simulink library "inp"  (R2021b)
settings: Solver=VariableStepAuto  StartTime=0.0  StopTime=10.0  RelTol=1e-3
undefined symbols (not defined in the file): C_TASK_5MS_S, FALSE, KINP_AcoreReadyToSlp_flg_ovrdflg, KINP_AcoreReadyToSlp_flg_ovrdval, KINP_AllowMovThd_OTA_enum_ovrdflg, KINP_AllowMovThd_OTA_enum_ovrdval, KINP_APSAngleTarget_Deg_ovrdflg, KINP_APSAngleTarget_Deg_ovrdval, KINP_APSDecReq_mps2_ovrdflg, KINP_APSDecReq_mps2_ovrdval, KINP_APSDecReqA_flg_ovrdflg, KINP_APSDecReqA_flg_ovrdval, KINP_APSDFLL_cm_ovrdflg, KINP_APSDFLL_cm_ovrdval, KINP_APSDFLR_cm_ovrdflg, KINP_APSDFLR_cm_ovrdval, KINP_APSDRLL_cm_ovrdflg, KINP_APSDRLL_cm_ovrdval, KINP_APSDRLR_cm_ovrdflg, KINP_APSDRLR_cm_ovrdval, KINP_APSExitCondition_enum_ovrdflg, KINP_APSExitCondition_enum_ovrdval, KINP_APSHWVer_enum_ovrdflg, KINP_APSHWVer_enum_ovrdval, KINP_APSProgressPCT_pct_ovrdflg, KINP_APSProgressPCT_pct_ovrdval, KINP_APSReq_enum_ovrdflg, KINP_APSReq_enum_ovrdval, KINP_APSRQDisplay_enum_ovrdflg, KINP_APSRQDisplay_enum_ovrdval, KINP_APSRqEPASCtrl_flg_ovrdflg, KINP_APSRqEPASCtrl_flg_ovrdval, KINP_APSShiftPosnReq_enum_ovrdval, KINP_APSShiftPosnReq_enum_ovrflg, KINP_APSSpeedCMD_kph_ovrdval, KINP_APSSpeedCMD_kph_ovrflg, KINP_APSStaSystem_enum_ovrdflg, KINP_APSStaSystem_enum_ovrdval, KINP_APSSWVer_enum_ovrdflg, KINP_APSSWVer_enum_ovrdval, KINP_APSVMCReqA_flg_ovrdval, KINP_APSVMCReqA_flg_ovrflg, KINP_APSVRqEPASCtrl_flg_ovrdflg, KINP_APSVRqEPASCtrl_flg_ovrdval, KINP_AuxBattVolmV_mV_ovrdflg, KINP_AuxBattVolmV_mV_ovrdval, KINP_CAASSta_enum_ovrdflg, KINP_CAASSta_enum_ovrdval, KINP_CAASVMCReqA_flg_ovrdval, KINP_CAASVMCReqA_flg_ovrflg, KINP_Chime_enum_ovrdflg, KINP_Chime_enum_ovrdval, KINP_ClearDTCcmd_flg_ovrdflg, KINP_ClearDTCcmd_flg_ovrdval, KINP_EvccAplusPwrUpReq_flg_ovrdflg, KINP_EvccAplusPwrUpReq_flg_ovrdval, KINP_LFID_raw_ovrdval, KINP_LFID_raw_ovrflg, KINP_LRID_raw_ovrdval, KINP_MemOffsetAccX_raw16_ovrdflg ... (+118)
libraries: FVT_lib x595, hcu_lib x1
(part 19 of 27)

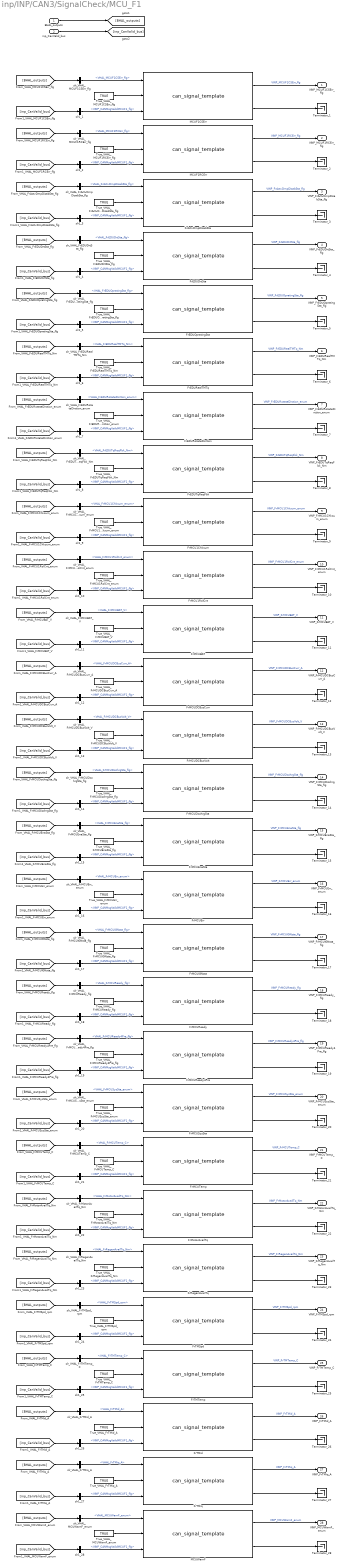
== system inp/INP/CAN3/SignalCheck/MCU_F1 ==
  BHAL_outputs : Inport
  inp_CanValid_bus : Inport  Port=2
  FrActvDmpDisabSta : FVT_lib/inp/can_signal_template  SystemSampleTime=-1  VariantActivationTime=update diagram  Latency=0  AutoFrameSizeCalculation=off
      link override defval: Value=KINP_FrActvDmpDisabSta_flg_defval
      link override fftdec: Value=KINP_FrActvDmpDisabSta_flg_fftdec
      link override fftinc: Value=KINP_FrActvDmpDisabSta_flg_fftinc
      link override fftlim: Value=KINP_FrActvDmpDisabSta_flg_fftlim
      link override invalid: Value=KINP_FrActvDmpDisabSta_flg_invalid
      link override ovrdflg: Value=KINP_FrActvDmpDisabSta_flg_ovrdflg
      link override ovrdval: Value=KINP_FrActvDmpDisabSta_flg_ovrdval
      link override setvalid: Value=KINP_FrActvDmpDisabSta_flg_setvalid
      link override srvcflg: Value=KINP_FrActvDmpDisabSta_flg_srvcflg
      link override srvcval: Value=KINP_FrActvDmpDisabSta_flg_srvcval
  FrEDUDrtSta : FVT_lib/inp/can_signal_template  SystemSampleTime=-1  VariantActivationTime=update diagram  Latency=0  AutoFrameSizeCalculation=off
      link override defval: Value=KINP_FrEDUDrtSta_flg_defval
      link override fftdec: Value=KINP_FrEDUDrtSta_flg_fftdec
      link override fftinc: Value=KINP_FrEDUDrtSta_flg_fftinc
      link override fftlim: Value=KINP_FrEDUDrtSta_flg_fftlim
      link override invalid: Value=KINP_FrEDUDrtSta_flg_invalid
      link override ovrdflg: Value=KINP_FrEDUDrtSta_flg_ovrdflg
      link override ovrdval: Value=KINP_FrEDUDrtSta_flg_ovrdval
      link override setvalid: Value=KINP_FrEDUDrtSta_flg_setvalid
      link override srvcflg: Value=KINP_FrEDUDrtSta_flg_srvcflg
      link override srvcval: Value=KINP_FrEDUDrtSta_flg_srvcval
  FrEDUOpratingSta : FVT_lib/inp/can_signal_template  SystemSampleTime=-1  VariantActivationTime=update diagram  Latency=0  AutoFrameSizeCalculation=off
      link override defval: Value=KINP_FrEDUOpratingSta_flg_defval
      link override fftdec: Value=KINP_FrEDUOpratingSta_flg_fftdec
      link override fftinc: Value=KINP_FrEDUOpratingSta_flg_fftinc
      link override fftlim: Value=KINP_FrEDUOpratingSta_flg_fftlim
      link override invalid: Value=KINP_FrEDUOpratingSta_flg_invalid
      link override ovrdflg: Value=KINP_FrEDUOpratingSta_flg_ovrdflg
      link override ovrdval: Value=KINP_FrEDUOpratingSta_flg_ovrdval
      link override setvalid: Value=KINP_FrEDUOpratingSta_flg_setvalid
      link override srvcflg: Value=KINP_FrEDUOpratingSta_flg_srvcflg
      link override srvcval: Value=KINP_FrEDUOpratingSta_flg_srvcval
  FrEDURealTMTq : FVT_lib/inp/can_signal_template  SystemSampleTime=-1  VariantActivationTime=update diagram  Latency=0  AutoFrameSizeCalculation=off
      link override defval: Value=KINP_FrEDURealTMTq_Nm_defval
      link override fftdec: Value=KINP_FrEDURealTMTq_Nm_fftdec
      link override fftinc: Value=KINP_FrEDURealTMTq_Nm_fftinc
      link override fftlim: Value=KINP_FrEDURealTMTq_Nm_fftlim
      link override invalid: Value=KINP_FrEDURealTMTq_Nm_invalid
      link override ovrdflg: Value=KINP_FrEDURealTMTq_Nm_ovrdflg
      link override ovrdval: Value=KINP_FrEDURealTMTq_Nm_ovrdval
      link override setvalid: Value=KINP_FrEDURealTMTq_Nm_setvalid
      link override srvcflg: Value=KINP_FrEDURealTMTq_Nm_srvcflg
      link override srvcval: Value=KINP_FrEDURealTMTq_Nm_srvcval
  FrEDURotateDirction : FVT_lib/inp/can_signal_template  SystemSampleTime=-1  VariantActivationTime=update diagram  Latency=0  AutoFrameSizeCalculation=off
      link override defval: Value=KINP_FrEDURotateDirction_enum_defval
      link override fftdec: Value=KINP_FrEDURotateDirction_enum_fftdec
      link override fftinc: Value=KINP_FrEDURotateDirction_enum_fftinc
      link override fftlim: Value=KINP_FrEDURotateDirction_enum_fftlim
      link override invalid: Value=KINP_FrEDURotateDirction_enum_invalid
      link override ovrdflg: Value=KINP_FrEDURotateDirction_enum_ovrdflg
      link override ovrdval: Value=KINP_FrEDURotateDirction_enum_ovrdval
      link override setvalid: Value=KINP_FrEDURotateDirction_enum_setvalid
      link override srvcflg: Value=KINP_FrEDURotateDirction_enum_srvcflg
      link override srvcval: Value=KINP_FrEDURotateDirction_enum_srvcval
  FrEDUTqReqFbk : FVT_lib/inp/can_signal_template  SystemSampleTime=-1  VariantActivationTime=update diagram  Latency=0  AutoFrameSizeCalculation=off
      link override defval: Value=KINP_FrEDUTqReqFbk_Nm_defval
      link override fftdec: Value=KINP_FrEDUTqReqFbk_Nm_fftdec
      link override fftinc: Value=KINP_FrEDUTqReqFbk_Nm_fftinc
      link override fftlim: Value=KINP_FrEDUTqReqFbk_Nm_fftlim
      link override invalid: Value=KINP_FrEDUTqReqFbk_Nm_invalid
      link override ovrdflg: Value=KINP_FrEDUTqReqFbk_Nm_ovrdflg
      link override ovrdval: Value=KINP_FrEDUTqReqFbk_Nm_ovrdval
      link override setvalid: Value=KINP_FrEDUTqReqFbk_Nm_setvalid
      link override srvcflg: Value=KINP_FrEDUTqReqFbk_Nm_srvcflg
      link override srvcval: Value=KINP_FrEDUTqReqFbk_Nm_srvcval
  FrMCU1Chksum : FVT_lib/inp/can_signal_template  SystemSampleTime=-1  VariantActivationTime=update diagram  Latency=0  AutoFrameSizeCalculation=off
      link override defval: Value=KINP_FrMCU1Chksum_enum_defval
      link override fftdec: Value=KINP_FrMCU1Chksum_enum_fftdec
      link override fftinc: Value=KINP_FrMCU1Chksum_enum_fftinc
      link override fftlim: Value=KINP_FrMCU1Chksum_enum_fftlim
      link override invalid: Value=KINP_FrMCU1Chksum_enum_invalid
      link override ovrdflg: Value=KINP_FrMCU1Chksum_enum_ovrdflg
      link override ovrdval: Value=KINP_FrMCU1Chksum_enum_ovrdval
      link override setvalid: Value=KINP_FrMCU1Chksum_enum_setvalid
      link override srvcflg: Value=KINP_FrMCU1Chksum_enum_srvcflg
      link override srvcval: Value=KINP_FrMCU1Chksum_enum_srvcval
  FrMCU1RolCnt : FVT_lib/inp/can_signal_template  SystemSampleTime=-1  VariantActivationTime=update diagram  Latency=0  AutoFrameSizeCalculation=off
      link override defval: Value=KINP_FrMCU1RolCnt_enum_defval
      link override fftdec: Value=KINP_FrMCU1RolCnt_enum_fftdec
      link override fftinc: Value=KINP_FrMCU1RolCnt_enum_fftinc
      link override fftlim: Value=KINP_FrMCU1RolCnt_enum_fftlim
      link override invalid: Value=KINP_FrMCU1RolCnt_enum_invalid
      link override ovrdflg: Value=KINP_FrMCU1RolCnt_enum_ovrdflg
      link override ovrdval: Value=KINP_FrMCU1RolCnt_enum_ovrdval
      link override setvalid: Value=KINP_FrMCU1RolCnt_enum_setvalid
      link override srvcflg: Value=KINP_FrMCU1RolCnt_enum_srvcflg
      link override srvcval: Value=KINP_FrMCU1RolCnt_enum_srvcval
  FrMCUBAT : FVT_lib/inp/can_signal_template  SystemSampleTime=-1  VariantActivationTime=update diagram  Latency=0  AutoFrameSizeCalculation=off
      link override defval: Value=KINP_FrMCUBAT_V_defval
      link override fftdec: Value=KINP_FrMCUBAT_V_fftdec
      link override fftinc: Value=KINP_FrMCUBAT_V_fftinc
      link override fftlim: Value=KINP_FrMCUBAT_V_fftlim
      link override invalid: Value=KINP_FrMCUBAT_V_invalid
      link override ovrdflg: Value=KINP_FrMCUBAT_V_ovrdflg
      link override ovrdval: Value=KINP_FrMCUBAT_V_ovrdval
      link override setvalid: Value=KINP_FrMCUBAT_V_setvalid
      link override srvcflg: Value=KINP_FrMCUBAT_V_srvcflg
      link override srvcval: Value=KINP_FrMCUBAT_V_srvcval
  FrMCUDCBusCurr : FVT_lib/inp/can_signal_template  SystemSampleTime=-1  VariantActivationTime=update diagram  Latency=0  AutoFrameSizeCalculation=off
      link override defval: Value=KINP_FrMCUDCBusCurr_A_defval
      link override fftdec: Value=KINP_FrMCUDCBusCurr_A_fftdec
      link override fftinc: Value=KINP_FrMCUDCBusCurr_A_fftinc
      link override fftlim: Value=KINP_FrMCUDCBusCurr_A_fftlim
      link override invalid: Value=KINP_FrMCUDCBusCurr_A_invalid
      link override ovrdflg: Value=KINP_FrMCUDCBusCurr_A_ovrdflg
      link override ovrdval: Value=KINP_FrMCUDCBusCurr_A_ovrdval
      link override setvalid: Value=KINP_FrMCUDCBusCurr_A_setvalid
      link override srvcflg: Value=KINP_FrMCUDCBusCurr_A_srvcflg
      link override srvcval: Value=KINP_FrMCUDCBusCurr_A_srvcval
  FrMCUDCBusVolt : FVT_lib/inp/can_signal_template  SystemSampleTime=-1  VariantActivationTime=update diagram  Latency=0  AutoFrameSizeCalculation=off
      link override defval: Value=KINP_FrMCUDCBusVolt_V_defval
      link override fftdec: Value=KINP_FrMCUDCBusVolt_V_fftdec
      link override fftinc: Value=KINP_FrMCUDCBusVolt_V_fftinc
      link override fftlim: Value=KINP_FrMCUDCBusVolt_V_fftlim
      link override invalid: Value=KINP_FrMCUDCBusVolt_V_invalid
      link override ovrdflg: Value=KINP_FrMCUDCBusVolt_V_ovrdflg
      link override ovrdval: Value=KINP_FrMCUDCBusVolt_V_ovrdval
      link override setvalid: Value=KINP_FrMCUDCBusVolt_V_setvalid
      link override srvcflg: Value=KINP_FrMCUDCBusVolt_V_srvcflg
      link override srvcval: Value=KINP_FrMCUDCBusVolt_V_srvcval
  FrMCUDischrgSta : FVT_lib/inp/can_signal_template  SystemSampleTime=-1  VariantActivationTime=update diagram  Latency=0  AutoFrameSizeCalculation=off
      link override defval: Value=KINP_FrMCUDischrgSta_flg_defval
      link override fftdec: Value=KINP_FrMCUDischrgSta_flg_fftdec
      link override fftinc: Value=KINP_FrMCUDischrgSta_flg_fftinc
      link override fftlim: Value=KINP_FrMCUDischrgSta_flg_fftlim
      link override invalid: Value=KINP_FrMCUDischrgSta_flg_invalid
      link override ovrdflg: Value=KINP_FrMCUDischrgSta_flg_ovrdflg
      link override ovrdval: Value=KINP_FrMCUDischrgSta_flg_ovrdval
      link override setvalid: Value=KINP_FrMCUDischrgSta_flg_setvalid
      link override srvcflg: Value=KINP_FrMCUDischrgSta_flg_srvcflg
      link override srvcval: Value=KINP_FrMCUDischrgSta_flg_srvcval
  FrMCUEnaSta : FVT_lib/inp/can_signal_template  SystemSampleTime=-1  VariantActivationTime=update diagram  Latency=0  AutoFrameSizeCalculation=off
      link override defval: Value=KINP_FrMCUEnaSta_flg_defval
      link override fftdec: Value=KINP_FrMCUEnaSta_flg_fftdec
      link override fftinc: Value=KINP_FrMCUEnaSta_flg_fftinc
      link override fftlim: Value=KINP_FrMCUEnaSta_flg_fftlim
      link override invalid: Value=KINP_FrMCUEnaSta_flg_invalid
      link override ovrdflg: Value=KINP_FrMCUEnaSta_flg_ovrdflg
      link override ovrdval: Value=KINP_FrMCUEnaSta_flg_ovrdval
      link override setvalid: Value=KINP_FrMCUEnaSta_flg_setvalid
      link override srvcflg: Value=KINP_FrMCUEnaSta_flg_srvcflg
      link override srvcval: Value=KINP_FrMCUEnaSta_flg_srvcval
  FrMCUErr : FVT_lib/inp/can_signal_template  SystemSampleTime=-1  VariantActivationTime=update diagram  Latency=0  AutoFrameSizeCalculation=off
      link override defval: Value=KINP_FrMCUErr_enum_defval
      link override fftdec: Value=KINP_FrMCUErr_enum_fftdec
      link override fftinc: Value=KINP_FrMCUErr_enum_fftinc
      link override fftlim: Value=KINP_FrMCUErr_enum_fftlim
      link override invalid: Value=KINP_FrMCUErr_enum_invalid
      link override ovrdflg: Value=KINP_FrMCUErr_enum_ovrdflg
      link override ovrdval: Value=KINP_FrMCUErr_enum_ovrdval
      link override setvalid: Value=KINP_FrMCUErr_enum_setvalid
      link override srvcflg: Value=KINP_FrMCUErr_enum_srvcflg
      link override srvcval: Value=KINP_FrMCUErr_enum_srvcval
  FrMCUIGNsta : FVT_lib/inp/can_signal_template  SystemSampleTime=-1  VariantActivationTime=update diagram  Latency=0  AutoFrameSizeCalculation=off
      link override defval: Value=KINP_FrMCUIGNsta_flg_defval
      link override fftdec: Value=KINP_FrMCUIGNsta_flg_fftdec
      link override fftinc: Value=KINP_FrMCUIGNsta_flg_fftinc
      link override fftlim: Value=KINP_FrMCUIGNsta_flg_fftlim
      link override invalid: Value=KINP_FrMCUIGNsta_flg_invalid
      link override ovrdflg: Value=KINP_FrMCUIGNsta_flg_ovrdflg
      link override ovrdval: Value=KINP_FrMCUIGNsta_flg_ovrdval
      link override setvalid: Value=KINP_FrMCUIGNsta_flg_setvalid
      link override srvcflg: Value=KINP_FrMCUIGNsta_flg_srvcflg
      link override srvcval: Value=KINP_FrMCUIGNsta_flg_srvcval
  FrMCUReady : FVT_lib/inp/can_signal_template  SystemSampleTime=-1  VariantActivationTime=update diagram  Latency=0  AutoFrameSizeCalculation=off
      link override defval: Value=KINP_FrMCUReady_flg_defval
      link override fftdec: Value=KINP_FrMCUReady_flg_fftdec
      link override fftinc: Value=KINP_FrMCUReady_flg_fftinc
      link override fftlim: Value=KINP_FrMCUReady_flg_fftlim
      link override invalid: Value=KINP_FrMCUReady_flg_invalid
      link override ovrdflg: Value=KINP_FrMCUReady_flg_ovrdflg
      link override ovrdval: Value=KINP_FrMCUReady_flg_ovrdval
      link override setvalid: Value=KINP_FrMCUReady_flg_setvalid
      link override srvcflg: Value=KINP_FrMCUReady_flg_srvcflg
      link override srvcval: Value=KINP_FrMCUReady_flg_srvcval
  FrMCUReady4Pre : FVT_lib/inp/can_signal_template  SystemSampleTime=-1  VariantActivationTime=update diagram  Latency=0  AutoFrameSizeCalculation=off
      link override defval: Value=KINP_FrMCUReady4Pre_flg_defval
      link override fftdec: Value=KINP_FrMCUReady4Pre_flg_fftdec
      link override fftinc: Value=KINP_FrMCUReady4Pre_flg_fftinc
      link override fftlim: Value=KINP_FrMCUReady4Pre_flg_fftlim
      link override invalid: Value=KINP_FrMCUReady4Pre_flg_invalid
      link override ovrdflg: Value=KINP_FrMCUReady4Pre_flg_ovrdflg
      link override ovrdval: Value=KINP_FrMCUReady4Pre_flg_ovrdval
      link override setvalid: Value=KINP_FrMCUReady4Pre_flg_setvalid
      link override srvcflg: Value=KINP_FrMCUReady4Pre_flg_srvcflg
      link override srvcval: Value=KINP_FrMCUReady4Pre_flg_srvcval
  FrMCUSysSta : FVT_lib/inp/can_signal_template  SystemSampleTime=-1  VariantActivationTime=update diagram  Latency=0  AutoFrameSizeCalculation=off
      link override defval: Value=KINP_FrMCUSysSta_enum_defval
      link override fftdec: Value=KINP_FrMCUSysSta_enum_fftdec
      link override fftinc: Value=KINP_FrMCUSysSta_enum_fftinc
      link override fftlim: Value=KINP_FrMCUSysSta_enum_fftlim
      link override invalid: Value=KINP_FrMCUSysSta_enum_invalid
      link override ovrdflg: Value=KINP_FrMCUSysSta_enum_ovrdflg
      link override ovrdval: Value=KINP_FrMCUSysSta_enum_ovrdval
      link override setvalid: Value=KINP_FrMCUSysSta_enum_setvalid
      link override srvcflg: Value=KINP_FrMCUSysSta_enum_srvcflg
      link override srvcval: Value=KINP_FrMCUSysSta_enum_srvcval
  FrMCUTemp : FVT_lib/inp/can_signal_template  SystemSampleTime=-1  VariantActivationTime=update diagram  Latency=0  AutoFrameSizeCalculation=off
      link override defval: Value=KINP_FrMCUTemp_C_defval
      link override fftdec: Value=KINP_FrMCUTemp_C_fftdec
      link override fftinc: Value=KINP_FrMCUTemp_C_fftinc
      link override fftlim: Value=KINP_FrMCUTemp_C_fftlim
      link override invalid: Value=KINP_FrMCUTemp_C_invalid
      link override ovrdflg: Value=KINP_FrMCUTemp_C_ovrdflg
      link override ovrdval: Value=KINP_FrMCUTemp_C_ovrdval
      link override setvalid: Value=KINP_FrMCUTemp_C_setvalid
      link override srvcflg: Value=KINP_FrMCUTemp_C_srvcflg
      link override srvcval: Value=KINP_FrMCUTemp_C_srvcval
  FrMotorAvailTq : FVT_lib/inp/can_signal_template  SystemSampleTime=-1  VariantActivationTime=update diagram  Latency=0  AutoFrameSizeCalculation=off
      link override defval: Value=KINP_FrMotorAvailTq_Nm_defval
      link override fftdec: Value=KINP_FrMotorAvailTq_Nm_fftdec
      link override fftinc: Value=KINP_FrMotorAvailTq_Nm_fftinc
      link override fftlim: Value=KINP_FrMotorAvailTq_Nm_fftlim
      link override invalid: Value=KINP_FrMotorAvailTq_Nm_invalid
      link override ovrdflg: Value=KINP_FrMotorAvailTq_Nm_ovrdflg
      link override ovrdval: Value=KINP_FrMotorAvailTq_Nm_ovrdval
      link override setvalid: Value=KINP_FrMotorAvailTq_Nm_setvalid
      link override srvcflg: Value=KINP_FrMotorAvailTq_Nm_srvcflg
      link override srvcval: Value=KINP_FrMotorAvailTq_Nm_srvcval
  FrRegenAvailTq : FVT_lib/inp/can_signal_template  SystemSampleTime=-1  VariantActivationTime=update diagram  Latency=0  AutoFrameSizeCalculation=off
      link override defval: Value=KINP_FrRegenAvailTq_Nm_defval
      link override fftdec: Value=KINP_FrRegenAvailTq_Nm_fftdec
      link override fftinc: Value=KINP_FrRegenAvailTq_Nm_fftinc
      link override fftlim: Value=KINP_FrRegenAvailTq_Nm_fftlim
      link override invalid: Value=KINP_FrRegenAvailTq_Nm_invalid
      link override ovrdflg: Value=KINP_FrRegenAvailTq_Nm_ovrdflg
      link override ovrdval: Value=KINP_FrRegenAvailTq_Nm_ovrdval
      link override setvalid: Value=KINP_FrRegenAvailTq_Nm_setvalid
      link override srvcflg: Value=KINP_FrRegenAvailTq_Nm_srvcflg
      link override srvcval: Value=KINP_FrRegenAvailTq_Nm_srvcval
  FrTMSpd : FVT_lib/inp/can_signal_template  SystemSampleTime=-1  VariantActivationTime=update diagram  Latency=0  AutoFrameSizeCalculation=off
      link override defval: Value=KINP_FrTMSpd_rpm_defval
      link override fftdec: Value=KINP_FrTMSpd_rpm_fftdec
      link override fftinc: Value=KINP_FrTMSpd_rpm_fftinc
      link override fftlim: Value=KINP_FrTMSpd_rpm_fftlim
      link override invalid: Value=KINP_FrTMSpd_rpm_invalid
      link override ovrdflg: Value=KINP_FrTMSpd_rpm_ovrdflg
      link override ovrdval: Value=KINP_FrTMSpd_rpm_ovrdval
      link override setvalid: Value=KINP_FrTMSpd_rpm_setvalid
      link override srvcflg: Value=KINP_FrTMSpd_rpm_srvcflg
      link override srvcval: Value=KINP_FrTMSpd_rpm_srvcval
  FrTMTemp : FVT_lib/inp/can_signal_template  SystemSampleTime=-1  VariantActivationTime=update diagram  Latency=0  AutoFrameSizeCalculation=off
      link override defval: Value=KINP_FrTMTemp_C_defval
      link override fftdec: Value=KINP_FrTMTemp_C_fftdec
      link override fftinc: Value=KINP_FrTMTemp_C_fftinc
      link override fftlim: Value=KINP_FrTMTemp_C_fftlim
      link override invalid: Value=KINP_FrTMTemp_C_invalid
      link override ovrdflg: Value=KINP_FrTMTemp_C_ovrdflg
      link override ovrdval: Value=KINP_FrTMTemp_C_ovrdval
      link override setvalid: Value=KINP_FrTMTemp_C_setvalid
      link override srvcflg: Value=KINP_FrTMTemp_C_srvcflg
      link override srvcval: Value=KINP_FrTMTemp_C_srvcval
  FrTMid : FVT_lib/inp/can_signal_template  SystemSampleTime=-1  VariantActivationTime=update diagram  Latency=0  AutoFrameSizeCalculation=off
      link override defval: Value=KINP_FrTMid_A_defval
      link override fftdec: Value=KINP_FrTMid_A_fftdec
      link override fftinc: Value=KINP_FrTMid_A_fftinc
      link override fftlim: Value=KINP_FrTMid_A_fftlim
      link override invalid: Value=KINP_FrTMid_A_invalid
      link override ovrdflg: Value=KINP_FrTMid_A_ovrdflg
      link override ovrdval: Value=KINP_FrTMid_A_ovrdval
      link override setvalid: Value=KINP_FrTMid_A_setvalid
      link override srvcflg: Value=KINP_FrTMid_A_srvcflg
      link override srvcval: Value=KINP_FrTMid_A_srvcval
  FrTMiq : FVT_lib/inp/can_signal_template  SystemSampleTime=-1  VariantActivationTime=update diagram  Latency=0  AutoFrameSizeCalculation=off
      link override defval: Value=KINP_FrTMiq_A_defval
      link override fftdec: Value=KINP_FrTMiq_A_fftdec
      link override fftinc: Value=KINP_FrTMiq_A_fftinc
      link override fftlim: Value=KINP_FrTMiq_A_fftlim
      link override invalid: Value=KINP_FrTMiq_A_invalid
      link override ovrdflg: Value=KINP_FrTMiq_A_ovrdflg
      link override ovrdval: Value=KINP_FrTMiq_A_ovrdval
      link override setvalid: Value=KINP_FrTMiq_A_setvalid
      link override srvcflg: Value=KINP_FrTMiq_A_srvcflg
      link override srvcval: Value=KINP_FrTMiq_A_srvcval
  MCUF1CSErr : FVT_lib/inp/can_signal_template  SystemSampleTime=-1  VariantActivationTime=update diagram  Latency=0  AutoFrameSizeCalculation=off
      link override defval: Value=KINP_MCUF1CSErr_flg_defval
      link override fftdec: Value=KINP_MCUF1CSErr_flg_fftdec
      link override fftinc: Value=KINP_MCUF1CSErr_flg_fftinc
      link override fftlim: Value=KINP_MCUF1CSErr_flg_fftlim
      link override invalid: Value=KINP_MCUF1CSErr_flg_invalid
      link override ovrdflg: Value=KINP_MCUF1CSErr_flg_ovrdflg
      link override ovrdval: Value=KINP_MCUF1CSErr_flg_ovrdval
      link override setvalid: Value=KINP_MCUF1CSErr_flg_setvalid
      link override srvcflg: Value=KINP_MCUF1CSErr_flg_srvcflg
      link override srvcval: Value=KINP_MCUF1CSErr_flg_srvcval
  MCUF1RCErr : FVT_lib/inp/can_signal_template  SystemSampleTime=-1  VariantActivationTime=update diagram  Latency=0  AutoFrameSizeCalculation=off
      link override defval: Value=KINP_MCUF1RCErr_flg_defval
      link override fftdec: Value=KINP_MCUF1RCErr_flg_fftdec
      link override fftinc: Value=KINP_MCUF1RCErr_flg_fftinc
      link override fftlim: Value=KINP_MCUF1RCErr_flg_fftlim
      link override invalid: Value=KINP_MCUF1RCErr_flg_invalid
      link override ovrdflg: Value=KINP_MCUF1RCErr_flg_ovrdflg
      link override ovrdval: Value=KINP_MCUF1RCErr_flg_ovrdval
      link override setvalid: Value=KINP_MCUF1RCErr_flg_setvalid
      link override srvcflg: Value=KINP_MCUF1RCErr_flg_srvcflg
      link override srvcval: Value=KINP_MCUF1RCErr_flg_srvcval
  MCUWarnF : FVT_lib/inp/can_signal_template  SystemSampleTime=-1  VariantActivationTime=update diagram  Latency=0  AutoFrameSizeCalculation=off
      link override defval: Value=KINP_MCUWarnF_enum_defval
      link override fftdec: Value=KINP_MCUWarnF_enum_fftdec
      link override fftinc: Value=KINP_MCUWarnF_enum_fftinc
      link override fftlim: Value=KINP_MCUWarnF_enum_fftlim
      link override invalid: Value=KINP_MCUWarnF_enum_invalid
      link override ovrdflg: Value=KINP_MCUWarnF_enum_ovrdflg
      link override ovrdval: Value=KINP_MCUWarnF_enum_ovrdval
      link override setvalid: Value=KINP_MCUWarnF_enum_setvalid
      link override srvcflg: Value=KINP_MCUWarnF_enum_srvcflg
      link override srvcval: Value=KINP_MCUWarnF_enum_srvcval
  Terminator_{1..28} (28 alike) : Terminator
  True_VHAL_FrActvDmpDisabSta_flg : Constant  Value=TRUE  OutDataTypeStr=boolean
  True_VHAL_FrEDUDrtSta_flg : Constant  Value=TRUE  OutDataTypeStr=boolean
  True_VHAL_FrEDUOpratingSta_flg : Constant  Value=TRUE  OutDataTypeStr=boolean
  True_VHAL_FrEDURealTMTq_Nm : Constant  Value=TRUE  OutDataTypeStr=boolean
  True_VHAL_FrEDURotateDirction_enum : Constant  Value=TRUE  OutDataTypeStr=boolean
  True_VHAL_FrEDUTqReqFbk_Nm : Constant  Value=TRUE  OutDataTypeStr=boolean
  True_VHAL_FrMCU1Chksum_enum : Constant  Value=TRUE  OutDataTypeStr=boolean
  True_VHAL_FrMCU1RolCnt_enum : Constant  Value=TRUE  OutDataTypeStr=boolean
  True_VHAL_FrMCUBAT_V : Constant  Value=TRUE  OutDataTypeStr=boolean
  True_VHAL_FrMCUDCBusCurr_A : Constant  Value=TRUE  OutDataTypeStr=boolean
  True_VHAL_FrMCUDCBusVolt_V : Constant  Value=TRUE  OutDataTypeStr=boolean
  True_VHAL_FrMCUDischrgSta_flg : Constant  Value=TRUE  OutDataTypeStr=boolean
  True_VHAL_FrMCUEnaSta_flg : Constant  Value=TRUE  OutDataTypeStr=boolean
  True_VHAL_FrMCUErr_enum : Constant  Value=TRUE  OutDataTypeStr=boolean
  True_VHAL_FrMCUIGNsta_flg : Constant  Value=TRUE  OutDataTypeStr=boolean
  True_VHAL_FrMCUReady4Pre_flg : Constant  Value=TRUE  OutDataTypeStr=boolean
  True_VHAL_FrMCUReady_flg : Constant  Value=TRUE  OutDataTypeStr=boolean
  True_VHAL_FrMCUSysSta_enum : Constant  Value=TRUE  OutDataTypeStr=boolean
  True_VHAL_FrMCUTemp_C : Constant  Value=TRUE  OutDataTypeStr=boolean
  True_VHAL_FrMotorAvailTq_Nm : Constant  Value=TRUE  OutDataTypeStr=boolean
  True_VHAL_FrRegenAvailTq_Nm : Constant  Value=TRUE  OutDataTypeStr=boolean
  True_VHAL_FrTMSpd_rpm : Constant  Value=TRUE  OutDataTypeStr=boolean
  True_VHAL_FrTMTemp_C : Constant  Value=TRUE  OutDataTypeStr=boolean
  True_VHAL_FrTMid_A : Constant  Value=TRUE  OutDataTypeStr=boolean
  True_VHAL_FrTMiq_A : Constant  Value=TRUE  OutDataTypeStr=boolean
  True_VHAL_MCUF1CSErr_flg : Constant  Value=TRUE  OutDataTypeStr=boolean
  True_VHAL_MCUF1RCErr_flg : Constant  Value=TRUE  OutDataTypeStr=boolean
  True_VHAL_MCUWarnF_enum : Constant  Value=TRUE  OutDataTypeStr=boolean
  slr1_{1..28} (28 alike) : BusSelector  OutputSignals=VINP_CANMsgValidMCUF1_flg
  slr_VHAL_FrActvDmpDisabSta_flg : BusSelector  OutputSignals=VHAL_FrActvDmpDisabSta_flg
  slr_VHAL_FrEDUDrtSta_flg : BusSelector  OutputSignals=VHAL_FrEDUDrtSta_flg
  slr_VHAL_FrEDUOpratingSta_flg : BusSelector  OutputSignals=VHAL_FrEDUOpratingSta_flg
  slr_VHAL_FrEDURealTMTq_Nm : BusSelector  OutputSignals=VHAL_FrEDURealTMTq_Nm
  slr_VHAL_FrEDURotateDirction_enum : BusSelector  OutputSignals=VHAL_FrEDURotateDirction_enum
  slr_VHAL_FrEDUTqReqFbk_Nm : BusSelector  OutputSignals=VHAL_FrEDUTqReqFbk_Nm
  slr_VHAL_FrMCU1Chksum_enum : BusSelector  OutputSignals=VHAL_FrMCU1Chksum_enum
  slr_VHAL_FrMCU1RolCnt_enum : BusSelector  OutputSignals=VHAL_FrMCU1RolCnt_enum
  slr_VHAL_FrMCUBAT_V : BusSelector  OutputSignals=VHAL_FrMCUBAT_V
  slr_VHAL_FrMCUDCBusCurr_A : BusSelector  OutputSignals=VHAL_FrMCUDCBusCurr_A
  slr_VHAL_FrMCUDCBusVolt_V : BusSelector  OutputSignals=VHAL_FrMCUDCBusVolt_V
  slr_VHAL_FrMCUDischrgSta_flg : BusSelector  OutputSignals=VHAL_FrMCUDischrgSta_flg
  slr_VHAL_FrMCUEnaSta_flg : BusSelector  OutputSignals=VHAL_FrMCUEnaSta_flg
  slr_VHAL_FrMCUErr_enum : BusSelector  OutputSignals=VHAL_FrMCUErr_enum
  slr_VHAL_FrMCUIGNsta_flg : BusSelector  OutputSignals=VHAL_FrMCUIGNsta_flg
  slr_VHAL_FrMCUReady4Pre_flg : BusSelector  OutputSignals=VHAL_FrMCUReady4Pre_flg
  slr_VHAL_FrMCUReady_flg : BusSelector  OutputSignals=VHAL_FrMCUReady_flg
  slr_VHAL_FrMCUSysSta_enum : BusSelector  OutputSignals=VHAL_FrMCUSysSta_enum
  slr_VHAL_FrMCUTemp_C : BusSelector  OutputSignals=VHAL_FrMCUTemp_C
  slr_VHAL_FrMotorAvailTq_Nm : BusSelector  OutputSignals=VHAL_FrMotorAvailTq_Nm
  slr_VHAL_FrRegenAvailTq_Nm : BusSelector  OutputSignals=VHAL_FrRegenAvailTq_Nm
  slr_VHAL_FrTMSpd_rpm : BusSelector  OutputSignals=VHAL_FrTMSpd_rpm
  slr_VHAL_FrTMTemp_C : BusSelector  OutputSignals=VHAL_FrTMTemp_C
  slr_VHAL_FrTMid_A : BusSelector  OutputSignals=VHAL_FrTMid_A
  slr_VHAL_FrTMiq_A : BusSelector  OutputSignals=VHAL_FrTMiq_A
  slr_VHAL_MCUF1CSErr_flg : BusSelector  OutputSignals=VHAL_MCUF1CSErr_flg
  slr_VHAL_MCUF1RCErr_flg : BusSelector  OutputSignals=VHAL_MCUF1RCErr_flg
  slr_VHAL_MCUWarnF_enum : BusSelector  OutputSignals=VHAL_MCUWarnF_enum
  VINP_MCUF1CSErr_flg : Outport
  VINP_MCUF1RCErr_flg : Outport  Port=2
  VINP_FrActvDmpDisabSta_flg : Outport  Port=3
  VINP_FrEDUDrtSta_flg : Outport  Port=4
  VINP_FrEDUOpratingSta_flg : Outport  Port=5
  VINP_FrEDURealTMTq_Nm : Outport  Port=6
  VINP_FrEDURotateDirction_enum : Outport  Port=7
  VINP_FrEDUTqReqFbk_Nm : Outport  Port=8
  VINP_FrMCU1Chksum_enum : Outport  Port=9
  VINP_FrMCU1RolCnt_enum : Outport  Port=10
  VINP_FrMCUBAT_V : Outport  Port=11
  VINP_FrMCUDCBusCurr_A : Outport  Port=12
  VINP_FrMCUDCBusVolt_V : Outport  Port=13
  VINP_FrMCUDischrgSta_flg : Outport  Port=14
  VINP_FrMCUEnaSta_flg : Outport  Port=15
  VINP_FrMCUErr_enum : Outport  Port=16
  VINP_FrMCUIGNsta_flg : Outport  Port=17
  VINP_FrMCUReady_flg : Outport  Port=18
  VINP_FrMCUReady4Pre_flg : Outport  Port=19
  VINP_FrMCUSysSta_enum : Outport  Port=20
  VINP_FrMCUTemp_C : Outport  Port=21
  VINP_FrMotorAvailTq_Nm : Outport  Port=22
  VINP_FrRegenAvailTq_Nm : Outport  Port=23
  VINP_FrTMSpd_rpm : Outport  Port=24
  VINP_FrTMTemp_C : Outport  Port=25
  VINP_FrTMid_A : Outport  Port=26
  VINP_FrTMiq_A : Outport  Port=27
  VINP_MCUWarnF_enum : Outport  Port=28
  wires:
  BHAL_outputs/1 -> [BHAL_outputs]
  inp_CanValid_bus/1 -> [inp_CanValid_bus]
  [BHAL_outputs] -> slr_VHAL_MCUF1CSErr_flg/1
  slr_VHAL_MCUF1CSErr_flg/1 -> MCUF1CSErr/1  "<VHAL_MCUF1CSErr_flg>"
  True_VHAL_MCUF1CSErr_flg/1 -> MCUF1CSErr/2
  [inp_CanValid_bus] -> slr1_1/1
  slr1_1/1 -> MCUF1CSErr/3  "<VINP_CANMsgValidMCUF1_flg>"
  MCUF1CSErr/1 -> VINP_MCUF1CSErr_flg/1  "VINP_MCUF1CSErr_flg"
  MCUF1CSErr/2 -> Terminator_1/1
  [BHAL_outputs] -> slr_VHAL_MCUF1RCErr_flg/1
  slr_VHAL_MCUF1RCErr_flg/1 -> MCUF1RCErr/1  "<VHAL_MCUF1RCErr_flg>"
  True_VHAL_MCUF1RCErr_flg/1 -> MCUF1RCErr/2
  [inp_CanValid_bus] -> slr1_2/1
  slr1_2/1 -> MCUF1RCErr/3  "<VINP_CANMsgValidMCUF1_flg>"
  MCUF1RCErr/1 -> VINP_MCUF1RCErr_flg/1  "VINP_MCUF1RCErr_flg"
  MCUF1RCErr/2 -> Terminator_2/1
  [BHAL_outputs] -> slr_VHAL_FrActvDmpDisabSta_flg/1
  slr_VHAL_FrActvDmpDisabSta_flg/1 -> FrActvDmpDisabSta/1  "<VHAL_FrActvDmpDisabSta_flg>"
  True_VHAL_FrActvDmpDisabSta_flg/1 -> FrActvDmpDisabSta/2
  [inp_CanValid_bus] -> slr1_3/1
  slr1_3/1 -> FrActvDmpDisabSta/3  "<VINP_CANMsgValidMCUF1_flg>"
  FrActvDmpDisabSta/1 -> VINP_FrActvDmpDisabSta_flg/1  "VINP_FrActvDmpDisabSta_flg"
  FrActvDmpDisabSta/2 -> Terminator_3/1
  [BHAL_outputs] -> slr_VHAL_FrEDUDrtSta_flg/1
  slr_VHAL_FrEDUDrtSta_flg/1 -> FrEDUDrtSta/1  "<VHAL_FrEDUDrtSta_flg>"
  True_VHAL_FrEDUDrtSta_flg/1 -> FrEDUDrtSta/2
  [inp_CanValid_bus] -> slr1_4/1
  slr1_4/1 -> FrEDUDrtSta/3  "<VINP_CANMsgValidMCUF1_flg>"
  FrEDUDrtSta/1 -> VINP_FrEDUDrtSta_flg/1  "VINP_FrEDUDrtSta_flg"
  FrEDUDrtSta/2 -> Terminator_4/1
  [BHAL_outputs] -> slr_VHAL_FrEDUOpratingSta_flg/1
  slr_VHAL_FrEDUOpratingSta_flg/1 -> FrEDUOpratingSta/1  "<VHAL_FrEDUOpratingSta_flg>"
  True_VHAL_FrEDUOpratingSta_flg/1 -> FrEDUOpratingSta/2
  [inp_CanValid_bus] -> slr1_5/1
  slr1_5/1 -> FrEDUOpratingSta/3  "<VINP_CANMsgValidMCUF1_flg>"
  FrEDUOpratingSta/1 -> VINP_FrEDUOpratingSta_flg/1  "VINP_FrEDUOpratingSta_flg"
  FrEDUOpratingSta/2 -> Terminator_5/1
  [BHAL_outputs] -> slr_VHAL_FrEDURealTMTq_Nm/1
  slr_VHAL_FrEDURealTMTq_Nm/1 -> FrEDURealTMTq/1  "<VHAL_FrEDURealTMTq_Nm>"
  True_VHAL_FrEDURealTMTq_Nm/1 -> FrEDURealTMTq/2
  [inp_CanValid_bus] -> slr1_6/1
  slr1_6/1 -> FrEDURealTMTq/3  "<VINP_CANMsgValidMCUF1_flg>"
  FrEDURealTMTq/1 -> VINP_FrEDURealTMTq_Nm/1  "VINP_FrEDURealTMTq_Nm"
  FrEDURealTMTq/2 -> Terminator_6/1
  [BHAL_outputs] -> slr_VHAL_FrEDURotateDirction_enum/1
  slr_VHAL_FrEDURotateDirction_enum/1 -> FrEDURotateDirction/1  "<VHAL_FrEDURotateDirction_enum>"
  True_VHAL_FrEDURotateDirction_enum/1 -> FrEDURotateDirction/2
  [inp_CanValid_bus] -> slr1_7/1
  slr1_7/1 -> FrEDURotateDirction/3  "<VINP_CANMsgValidMCUF1_flg>"
  FrEDURotateDirction/1 -> VINP_FrEDURotateDirction_enum/1  "VINP_FrEDURotateDirction_enum"
  FrEDURotateDirction/2 -> Terminator_7/1
  [BHAL_outputs] -> slr_VHAL_FrEDUTqReqFbk_Nm/1
  slr_VHAL_FrEDUTqReqFbk_Nm/1 -> FrEDUTqReqFbk/1  "<VHAL_FrEDUTqReqFbk_Nm>"
  True_VHAL_FrEDUTqReqFbk_Nm/1 -> FrEDUTqReqFbk/2
  [inp_CanValid_bus] -> slr1_8/1
  slr1_8/1 -> FrEDUTqReqFbk/3  "<VINP_CANMsgValidMCUF1_flg>"
  FrEDUTqReqFbk/1 -> VINP_FrEDUTqReqFbk_Nm/1  "VINP_FrEDUTqReqFbk_Nm"
  FrEDUTqReqFbk/2 -> Terminator_8/1
  [BHAL_outputs] -> slr_VHAL_FrMCU1Chksum_enum/1
  slr_VHAL_FrMCU1Chksum_enum/1 -> FrMCU1Chksum/1  "<VHAL_FrMCU1Chksum_enum>"
  True_VHAL_FrMCU1Chksum_enum/1 -> FrMCU1Chksum/2
  [inp_CanValid_bus] -> slr1_9/1
  slr1_9/1 -> FrMCU1Chksum/3  "<VINP_CANMsgValidMCUF1_flg>"
  FrMCU1Chksum/1 -> VINP_FrMCU1Chksum_enum/1  "VINP_FrMCU1Chksum_enum"
  FrMCU1Chksum/2 -> Terminator_9/1
  [BHAL_outputs] -> slr_VHAL_FrMCU1RolCnt_enum/1
  slr_VHAL_FrMCU1RolCnt_enum/1 -> FrMCU1RolCnt/1  "<VHAL_FrMCU1RolCnt_enum>"
  True_VHAL_FrMCU1RolCnt_enum/1 -> FrMCU1RolCnt/2
  [inp_CanValid_bus] -> slr1_10/1
  slr1_10/1 -> FrMCU1RolCnt/3  "<VINP_CANMsgValidMCUF1_flg>"
  FrMCU1RolCnt/1 -> VINP_FrMCU1RolCnt_enum/1  "VINP_FrMCU1RolCnt_enum"
  FrMCU1RolCnt/2 -> Terminator_10/1
  [BHAL_outputs] -> slr_VHAL_FrMCUBAT_V/1
  slr_VHAL_FrMCUBAT_V/1 -> FrMCUBAT/1  "<VHAL_FrMCUBAT_V>"
  True_VHAL_FrMCUBAT_V/1 -> FrMCUBAT/2
  [inp_CanValid_bus] -> slr1_11/1
  slr1_11/1 -> FrMCUBAT/3  "<VINP_CANMsgValidMCUF1_flg>"
  FrMCUBAT/1 -> VINP_FrMCUBAT_V/1  "VINP_FrMCUBAT_V"
  FrMCUBAT/2 -> Terminator_11/1
  [BHAL_outputs] -> slr_VHAL_FrMCUDCBusCurr_A/1
  slr_VHAL_FrMCUDCBusCurr_A/1 -> FrMCUDCBusCurr/1  "<VHAL_FrMCUDCBusCurr_A>"
  True_VHAL_FrMCUDCBusCurr_A/1 -> FrMCUDCBusCurr/2
  [inp_CanValid_bus] -> slr1_12/1
  slr1_12/1 -> FrMCUDCBusCurr/3  "<VINP_CANMsgValidMCUF1_flg>"
  FrMCUDCBusCurr/1 -> VINP_FrMCUDCBusCurr_A/1  "VINP_FrMCUDCBusCurr_A"
  FrMCUDCBusCurr/2 -> Terminator_12/1
  [BHAL_outputs] -> slr_VHAL_FrMCUDCBusVolt_V/1
  slr_VHAL_FrMCUDCBusVolt_V/1 -> FrMCUDCBusVolt/1  "<VHAL_FrMCUDCBusVolt_V>"
  True_VHAL_FrMCUDCBusVolt_V/1 -> FrMCUDCBusVolt/2
  [inp_CanValid_bus] -> slr1_13/1
  slr1_13/1 -> FrMCUDCBusVolt/3  "<VINP_CANMsgValidMCUF1_flg>"
  FrMCUDCBusVolt/1 -> VINP_FrMCUDCBusVolt_V/1  "VINP_FrMCUDCBusVolt_V"
  FrMCUDCBusVolt/2 -> Terminator_13/1
  [BHAL_outputs] -> slr_VHAL_FrMCUDischrgSta_flg/1
  slr_VHAL_FrMCUDischrgSta_flg/1 -> FrMCUDischrgSta/1  "<VHAL_FrMCUDischrgSta_flg>"
  True_VHAL_FrMCUDischrgSta_flg/1 -> FrMCUDischrgSta/2
  [inp_CanValid_bus] -> slr1_14/1
  slr1_14/1 -> FrMCUDischrgSta/3  "<VINP_CANMsgValidMCUF1_flg>"
  FrMCUDischrgSta/1 -> VINP_FrMCUDischrgSta_flg/1  "VINP_FrMCUDischrgSta_flg"
  FrMCUDischrgSta/2 -> Terminator_14/1
  [BHAL_outputs] -> slr_VHAL_FrMCUEnaSta_flg/1
  slr_VHAL_FrMCUEnaSta_flg/1 -> FrMCUEnaSta/1  "<VHAL_FrMCUEnaSta_flg>"
  True_VHAL_FrMCUEnaSta_flg/1 -> FrMCUEnaSta/2
  [inp_CanValid_bus] -> slr1_15/1
  slr1_15/1 -> FrMCUEnaSta/3  "<VINP_CANMsgValidMCUF1_flg>"
  FrMCUEnaSta/1 -> VINP_FrMCUEnaSta_flg/1  "VINP_FrMCUEnaSta_flg"
  FrMCUEnaSta/2 -> Terminator_15/1
  [BHAL_outputs] -> slr_VHAL_FrMCUErr_enum/1
  slr_VHAL_FrMCUErr_enum/1 -> FrMCUErr/1  "<VHAL_FrMCUErr_enum>"
  True_VHAL_FrMCUErr_enum/1 -> FrMCUErr/2
  [inp_CanValid_bus] -> slr1_16/1
  slr1_16/1 -> FrMCUErr/3  "<VINP_CANMsgValidMCUF1_flg>"
  FrMCUErr/1 -> VINP_FrMCUErr_enum/1  "VINP_FrMCUErr_enum"
  FrMCUErr/2 -> Terminator_16/1
  [BHAL_outputs] -> slr_VHAL_FrMCUIGNsta_flg/1
  slr_VHAL_FrMCUIGNsta_flg/1 -> FrMCUIGNsta/1  "<VHAL_FrMCUIGNsta_flg>"
  True_VHAL_FrMCUIGNsta_flg/1 -> FrMCUIGNsta/2
  [inp_CanValid_bus] -> slr1_17/1
  slr1_17/1 -> FrMCUIGNsta/3  "<VINP_CANMsgValidMCUF1_flg>"
  FrMCUIGNsta/1 -> VINP_FrMCUIGNsta_flg/1  "VINP_FrMCUIGNsta_flg"
  FrMCUIGNsta/2 -> Terminator_17/1
  [BHAL_outputs] -> slr_VHAL_FrMCUReady_flg/1
  slr_VHAL_FrMCUReady_flg/1 -> FrMCUReady/1  "<VHAL_FrMCUReady_flg>"
  True_VHAL_FrMCUReady_flg/1 -> FrMCUReady/2
  [inp_CanValid_bus] -> slr1_18/1
  slr1_18/1 -> FrMCUReady/3  "<VINP_CANMsgValidMCUF1_flg>"
  FrMCUReady/1 -> VINP_FrMCUReady_flg/1  "VINP_FrMCUReady_flg"
  FrMCUReady/2 -> Terminator_18/1
  [BHAL_outputs] -> slr_VHAL_FrMCUReady4Pre_flg/1
  slr_VHAL_FrMCUReady4Pre_flg/1 -> FrMCUReady4Pre/1  "<VHAL_FrMCUReady4Pre_flg>"
  True_VHAL_FrMCUReady4Pre_flg/1 -> FrMCUReady4Pre/2
  [inp_CanValid_bus] -> slr1_19/1
  slr1_19/1 -> FrMCUReady4Pre/3  "<VINP_CANMsgValidMCUF1_flg>"
  FrMCUReady4Pre/1 -> VINP_FrMCUReady4Pre_flg/1  "VINP_FrMCUReady4Pre_flg"
  FrMCUReady4Pre/2 -> Terminator_19/1
  [BHAL_outputs] -> slr_VHAL_FrMCUSysSta_enum/1
  slr_VHAL_FrMCUSysSta_enum/1 -> FrMCUSysSta/1  "<VHAL_FrMCUSysSta_enum>"
  True_VHAL_FrMCUSysSta_enum/1 -> FrMCUSysSta/2
  [inp_CanValid_bus] -> slr1_20/1
  slr1_20/1 -> FrMCUSysSta/3  "<VINP_CANMsgValidMCUF1_flg>"
  FrMCUSysSta/1 -> VINP_FrMCUSysSta_enum/1  "VINP_FrMCUSysSta_enum"
  FrMCUSysSta/2 -> Terminator_20/1
  [BHAL_outputs] -> slr_VHAL_FrMCUTemp_C/1
  slr_VHAL_FrMCUTemp_C/1 -> FrMCUTemp/1  "<VHAL_FrMCUTemp_C>"
  True_VHAL_FrMCUTemp_C/1 -> FrMCUTemp/2
  [inp_CanValid_bus] -> slr1_21/1
  slr1_21/1 -> FrMCUTemp/3  "<VINP_CANMsgValidMCUF1_flg>"
  FrMCUTemp/1 -> VINP_FrMCUTemp_C/1  "VINP_FrMCUTemp_C"
  FrMCUTemp/2 -> Terminator_21/1
  [BHAL_outputs] -> slr_VHAL_FrMotorAvailTq_Nm/1
  slr_VHAL_FrMotorAvailTq_Nm/1 -> FrMotorAvailTq/1  "<VHAL_FrMotorAvailTq_Nm>"
  True_VHAL_FrMotorAvailTq_Nm/1 -> FrMotorAvailTq/2
  [inp_CanValid_bus] -> slr1_22/1
  slr1_22/1 -> FrMotorAvailTq/3  "<VINP_CANMsgValidMCUF1_flg>"
  FrMotorAvailTq/1 -> VINP_FrMotorAvailTq_Nm/1  "VINP_FrMotorAvailTq_Nm"
  FrMotorAvailTq/2 -> Terminator_22/1
  [BHAL_outputs] -> slr_VHAL_FrRegenAvailTq_Nm/1
  slr_VHAL_FrRegenAvailTq_Nm/1 -> FrRegenAvailTq/1  "<VHAL_FrRegenAvailTq_Nm>"
  True_VHAL_FrRegenAvailTq_Nm/1 -> FrRegenAvailTq/2
  [inp_CanValid_bus] -> slr1_23/1
  slr1_23/1 -> FrRegenAvailTq/3  "<VINP_CANMsgValidMCUF1_flg>"
  FrRegenAvailTq/1 -> VINP_FrRegenAvailTq_Nm/1  "VINP_FrRegenAvailTq_Nm"
  FrRegenAvailTq/2 -> Terminator_23/1
  [BHAL_outputs] -> slr_VHAL_FrTMSpd_rpm/1
  slr_VHAL_FrTMSpd_rpm/1 -> FrTMSpd/1  "<VHAL_FrTMSpd_rpm>"
  True_VHAL_FrTMSpd_rpm/1 -> FrTMSpd/2
  [inp_CanValid_bus] -> slr1_24/1
  slr1_24/1 -> FrTMSpd/3  "<VINP_CANMsgValidMCUF1_flg>"
  FrTMSpd/1 -> VINP_FrTMSpd_rpm/1  "VINP_FrTMSpd_rpm"
  FrTMSpd/2 -> Terminator_24/1
  [BHAL_outputs] -> slr_VHAL_FrTMTemp_C/1
  slr_VHAL_FrTMTemp_C/1 -> FrTMTemp/1  "<VHAL_FrTMTemp_C>"
  True_VHAL_FrTMTemp_C/1 -> FrTMTemp/2
  [inp_CanValid_bus] -> slr1_25/1
  slr1_25/1 -> FrTMTemp/3  "<VINP_CANMsgValidMCUF1_flg>"
  FrTMTemp/1 -> VINP_FrTMTemp_C/1  "VINP_FrTMTemp_C"
  FrTMTemp/2 -> Terminator_25/1
  [BHAL_outputs] -> slr_VHAL_FrTMid_A/1
  slr_VHAL_FrTMid_A/1 -> FrTMid/1  "<VHAL_FrTMid_A>"
  True_VHAL_FrTMid_A/1 -> FrTMid/2
  [inp_CanValid_bus] -> slr1_26/1
  slr1_26/1 -> FrTMid/3  "<VINP_CANMsgValidMCUF1_flg>"
  FrTMid/1 -> VINP_FrTMid_A/1  "VINP_FrTMid_A"
  FrTMid/2 -> Terminator_26/1
  [BHAL_outputs] -> slr_VHAL_FrTMiq_A/1
  slr_VHAL_FrTMiq_A/1 -> FrTMiq/1  "<VHAL_FrTMiq_A>"
  True_VHAL_FrTMiq_A/1 -> FrTMiq/2
  [inp_CanValid_bus] -> slr1_27/1
  slr1_27/1 -> FrTMiq/3  "<VINP_CANMsgValidMCUF1_flg>"
  FrTMiq/1 -> VINP_FrTMiq_A/1  "VINP_FrTMiq_A"
  FrTMiq/2 -> Terminator_27/1
  [BHAL_outputs] -> slr_VHAL_MCUWarnF_enum/1
  slr_VHAL_MCUWarnF_enum/1 -> MCUWarnF/1  "<VHAL_MCUWarnF_enum>"
  True_VHAL_MCUWarnF_enum/1 -> MCUWarnF/2
  [inp_CanValid_bus] -> slr1_28/1
  slr1_28/1 -> MCUWarnF/3  "<VINP_CANMsgValidMCUF1_flg>"
  MCUWarnF/1 -> VINP_MCUWarnF_enum/1  "VINP_MCUWarnF_enum"
  MCUWarnF/2 -> Terminator_28/1
